simulink model "p2"  (R2020a)
settings: Solver=VariableStepAuto  StartTime=0.0  StopTime=10.0  RelTol=1e-3
model workspace (MAT data in the model file):
  b = Simulink.Parameter
  b.Value = 1
  b.DataType = 'auto'
  b.Dimensions = [1 1]
  k = Simulink.Parameter
  k.Value = 1
  k.DataType = 'auto'
  k.Dimensions = [1 1]
  k1 = Simulink.Parameter
  k1.Value = 1
  k1.DataType = 'auto'
  k1.Dimensions = [1 1]
  k2 = Simulink.Parameter
  k2.Value = 1
  k2.DataType = 'auto'
  k2.Dimensions = [1 1]
settings Model: Creator=007  LastModifiedBy=007

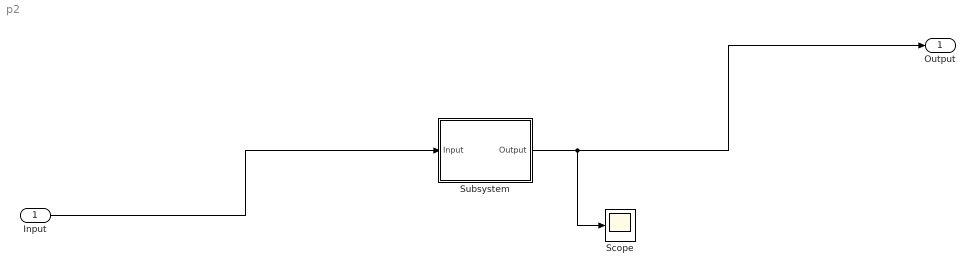
== system p2 ==
  Input : Inport
  Scope : Scope
  Subsystem : Subsystem
  Output : Outport
  wires:
  Input/1 -> Subsystem/1(Input)
  Subsystem/1(Output) -> Scope/1, Output/1

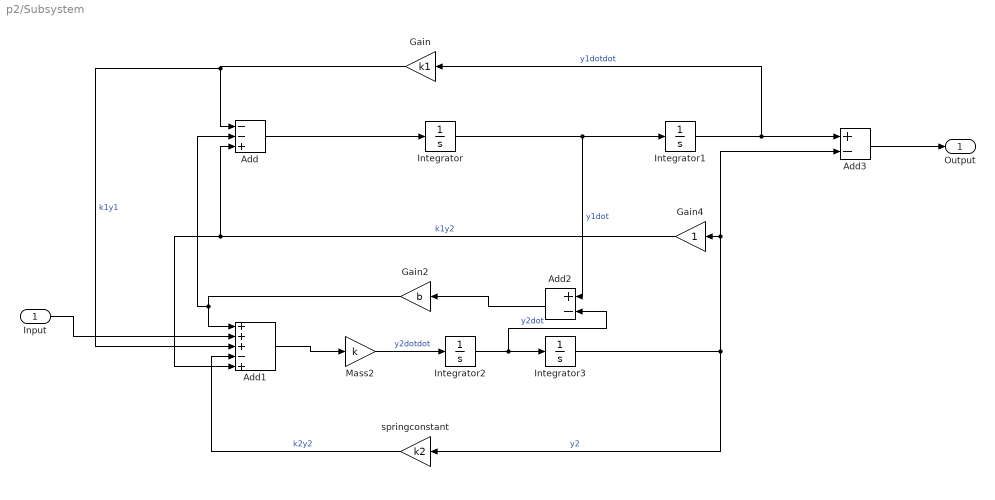
== system p2/Subsystem ==
  Input : Inport
  Add : Sum  Inputs=--+
  Add1 : Sum  Inputs=+++-+
  Add2 : Sum  Inputs=+-
  Add3 : Sum  Inputs=+-
  Gain : Gain  Gain=k1
  Gain2 : Gain  Gain=b
  Gain4 : Gain
  Integrator{,1..3} (4 alike) : Integrator
  Mass2 : Gain  Gain=k
  springconstant : Gain  Gain=k2
  Output : Outport
  wires:
  Integrator2/1 -> Add2/2, Integrator3/1  "y2dot"
  Gain4/1 -> Add1/5, Add/3  "k1y2"
  Add/1 -> Integrator/1
  Add3/1 -> Output/1
  Integrator/1 -> Add2/1, Integrator1/1  "y1dot"
  Add1/1 -> Mass2/1
  Integrator1/1 -> Gain/1, Add3/1  "y1dotdot"
  Integrator3/1 -> springconstant/1, Add3/2, Gain4/1  "y2"
  Gain/1 -> Add1/3, Add/1  "k1y1"
  Mass2/1 -> Integrator2/1  "y2dotdot"
  Add2/1 -> Gain2/1
  Input/1 -> Add1/2
  Gain2/1 -> Add1/1, Add/2
  springconstant/1 -> Add1/4  "k2y2"
